simulink model "Step_response"  (R2021a)
settings: Solver=VariableStepAuto  StartTime=0.0  StopTime=10.0  RelTol=1e-3
values from neighbouring files (symbols this model uses):
  b = .5    (= 0.5)    [RunStep_response.m]    (also in Runmotorsim.m)
  J = .05    (= 0.05)    [RunStep_response.m]    (also in Runmotorsim.m)
  Ke = .5    (= 0.5)    [RunStep_response.m]    (also in Runmotorsim.m)
  Kt = 1    [RunStep_response.m]    (also in Runmotorsim.m = 0.5)
  Ra = 1    [RunStep_response.m]    (also in Runmotorsim.m)
settings Model: Creator=Beau Collins  LastModifiedBy=abcollins
settings SolverCC: AlgebraicLoopSolver=TrustRegion
settings DebuggingCC: SFMachineParentedDataDiag=warning

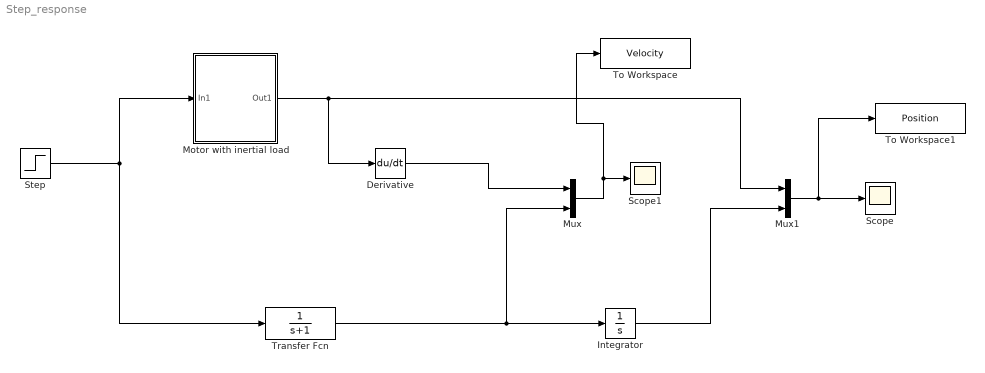
== system Step_response ==
  Derivative : Derivative
  Integrator : Integrator
  Motor with inertial load : Subsystem
  Mux : Mux  Inputs=2
  Mux1 : Mux  Inputs=2
  Scope : Scope
  Scope1 : Scope
  Step : Step  SampleTime=0
  To Workspace : ToWorkspace  VariableName=Velocity  SaveFormat=Timeseries  SampleTime=-1
  To Workspace1 : ToWorkspace  VariableName=Position  SaveFormat=Timeseries  SampleTime=-1
  Transfer Fcn : TransferFcn  Denominator=[1 1]
  wires:
  Step/1 -> Transfer Fcn/1, Motor with inertial load/1(In1)
  Motor with inertial load/1(Out1) -> Mux1/1, Derivative/1
  Derivative/1 -> Mux/1
  Transfer Fcn/1 -> Mux/2, Integrator/1
  Mux/1 -> To Workspace/1, Scope1/1
  Mux1/1 -> To Workspace1/1, Scope/1
  Integrator/1 -> Mux1/2

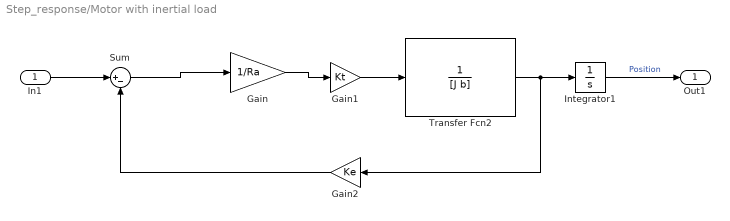
== system Step_response/Motor with inertial load ==
  In1 : Inport
  Gain : Gain  Gain=1/Ra
  Gain1 : Gain  Gain=Kt
  Gain2 : Gain  Gain=Ke
  Integrator1 : Integrator
  Sum : Sum  Inputs=|+-
  Transfer Fcn2 : TransferFcn  Denominator=[J b]  ContinuousStateAttributes='Transfer_Fcn'
  Out1 : Outport
  wires:
  Gain2/1 -> Sum/2
  Gain/1 -> Gain1/1
  Transfer Fcn2/1 -> Gain2/1, Integrator1/1
  In1/1 -> Sum/1
  Integrator1/1 -> Out1/1  "Position"
  Sum/1 -> Gain/1
  Gain1/1 -> Transfer Fcn2/1
